simulink model "Ex6_Coupled_ODE_ver1"  (R2020b)
settings: Solver=VariableStepAuto  StartTime=0.0  StopTime=5  RelTol=1e-3
settings Model: Creator=sulay  LastModifiedBy=sulay

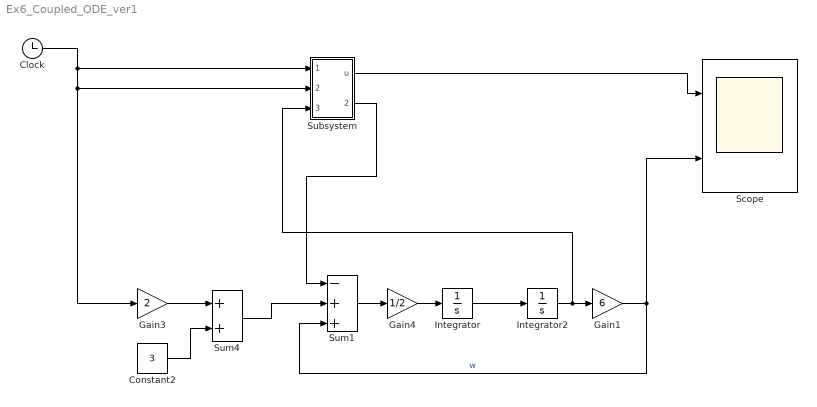
== system Ex6_Coupled_ODE_ver1 ==
  Clock : Clock
  Constant2 : Constant  Value=3
  Gain1 : Gain  Gain=6
  Gain3 : Gain  Gain=2
  Gain4 : Gain  Gain=1/2
  Integrator : Integrator  InitialCondition=4
  Integrator2 : Integrator  InitialCondition=3
  Scope : Scope  NumInputPorts=2
  Subsystem : Subsystem
  Sum1 : Sum  Inputs=-++
  Sum4 : Sum
  wires:
  Sum1/1 -> Gain4/1
  Integrator/1 -> Integrator2/1
  Integrator2/1 -> Subsystem/3(In3), Gain1/1
  Clock/1 -> Subsystem/1(In1), Gain3/1, Subsystem/2(In2)
  Gain1/1 -> Scope/2, Sum1/3  "w"
  Gain3/1 -> Sum4/1
  Constant2/1 -> Sum4/2
  Sum4/1 -> Sum1/2
  Gain4/1 -> Integrator/1
  Subsystem/1(u) -> Scope/1
  Subsystem/2(Out2) -> Sum1/1

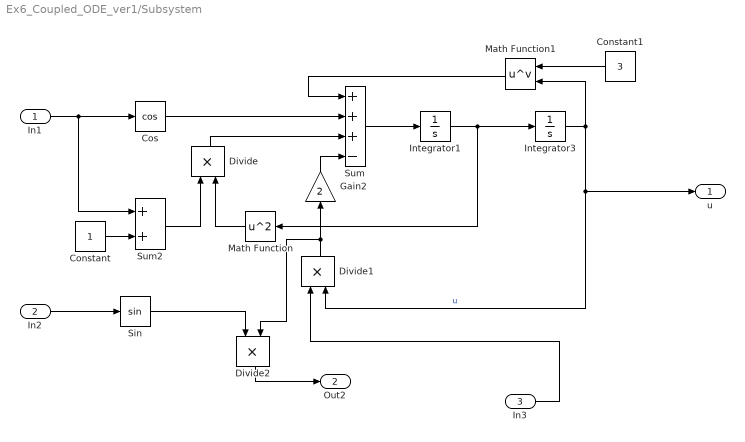
== system Ex6_Coupled_ODE_ver1/Subsystem ==
  In1 : Inport
  In2 : Inport  Port=2
  In3 : Inport  Port=3
  Constant : Constant
  Constant1 : Constant  Value=3
  Cos : Trigonometry  Operator=cos
  Divide : Product  Inputs=**
  Divide1 : Product  Inputs=**
  Divide2 : Product  Inputs=**
  Gain2 : Gain  Gain=2
  Integrator1 : Integrator  InitialCondition=2
  Integrator3 : Integrator  InitialCondition=1
  Math Function : Math  Operator=square  SaturateOnIntegerOverflow=on
  Math Function1 : Math  Operator=pow  SaturateOnIntegerOverflow=on
  Sin : Trigonometry
  Sum : Sum  Inputs=+++-
  Sum2 : Sum
  u : Outport
  Out2 : Outport  Port=2
  wires:
  Sum2/1 -> Divide/1
  Constant/1 -> Sum2/2
  Constant1/1 -> Math Function1/1
  Cos/1 -> Sum/2
  In2/1 -> Sin/1
  Math Function/1 -> Divide/2
  In1/1 -> Sum2/1, Cos/1
  Sum/1 -> Integrator1/1
  Gain2/1 -> Sum/4
  Divide1/1 -> Gain2/1, Divide2/2
  Integrator3/1 -> u/1, Divide1/2, Math Function1/2  "u"
  Integrator1/1 -> Integrator3/1, Math Function/1
  Sin/1 -> Divide2/1
  Divide2/1 -> Out2/1
  Divide/1 -> Sum/3
  Math Function1/1 -> Sum/1
  In3/1 -> Divide1/1
